simulink model "AutoRS_Simulation"  (R2022b)
settings: Solver=FixedStepAuto  StartTime=0.0  StopTime=350  FixedStep=1/10e3  RelTol=1e-3
undefined symbols (not defined in the file): beta_array, CQ_entries, CT_entries, d_B, d_T, k_B, k_T, lambda_array, m_B, m_T, param_const, param_opt
settings Model: Creator=Aaron  LastModifiedBy=Sebastian
settings DebuggingCC: UnconnectedInputMsg=warning  UnconnectedOutputMsg=warning  UnconnectedLineMsg=warning
settings ModelReferenceCC: EnableRefExpFcnMdlSchedulingChecks=on
settings RTWCC: DLArmComputeVersion=19.05

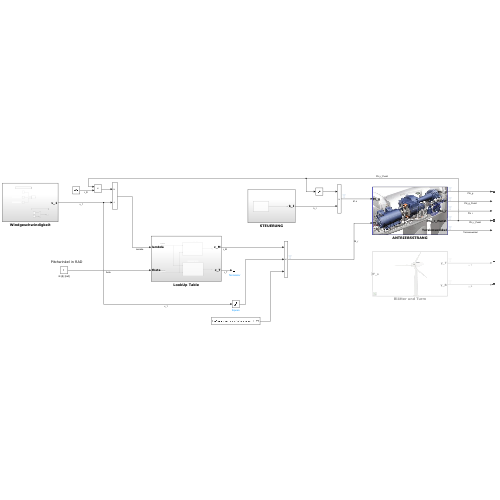
[thumbnail: Simulink's stored preview of the top-level diagram]
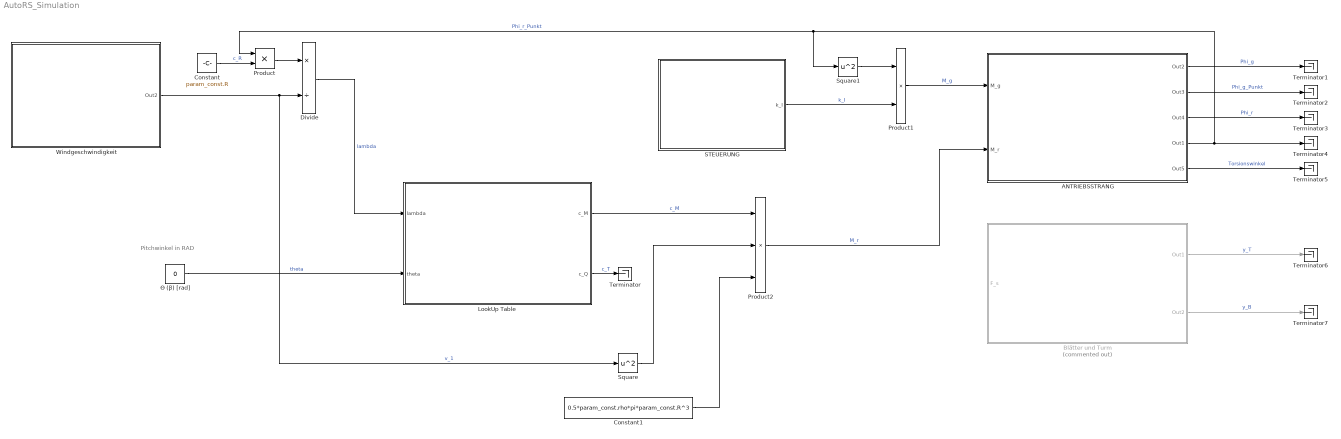
== system AutoRS_Simulation ==
  note: Pitchwinkel in RAD
  ANTRIEBSSTRANG : Subsystem
      mask Display: image('$imagefile'); % Use "Edit Image" on toolstrip to change.
  Blätter und Turm : Subsystem  Commented=on
      mask Display: image('$imagefile'); % Use "Edit Image" on toolstrip to change.
  Constant : Constant  Value=param_const.R
  Constant1 : Constant  Value=0.5*param_const.rho*pi*param_const.R^3
  Divide : Product  Inputs=*/
  LookUp Table : Subsystem
  Product : Product
  Product1 : Product
  Product2 : Product  Inputs=3
  STEUERUNG : Subsystem
  Square : Math  Operator=square
  Square1 : Math  Operator=square
  Terminator{,1..7} (8 alike) : Terminator
  Windgeschwindigkeit : Subsystem
  Θ (β) [rad] : Constant  Value=0
  wires:
  Divide/1 -> LookUp Table/1(lambda)  "lambda"
  Θ (β) [rad]/1 -> LookUp Table/2(theta)  "theta"
  ANTRIEBSSTRANG/1(Out2) -> Terminator1/1  "Phi_g"
  ANTRIEBSSTRANG/2(Out3) -> Terminator2/1  "Phi_g_Punkt"
  ANTRIEBSSTRANG/3(Out4) -> Terminator3/1  "Phi_r"
  ANTRIEBSSTRANG/4(Out1) -> Square1/1, Product/1, Terminator4/1  "Phi_r_Punkt"
  ANTRIEBSSTRANG/5(Out5) -> Terminator5/1  "Torsionswinkel"
  Blätter und Turm/1(Out1) -> Terminator6/1  "y_T"
  Blätter und Turm/2(Out2) -> Terminator7/1  "y_B"
  Product/1 -> Divide/1
  Constant/1 -> Product/2  "c_R"
  Windgeschwindigkeit/1(Out2) -> Square/1, Divide/2  "v_1"
  Product1/1 -> ANTRIEBSSTRANG/1(M_g)  "M_g"
  Product2/1 -> ANTRIEBSSTRANG/2(M_r)  "M_r"
  Square1/1 -> Product1/1
  LookUp Table/2(c_Q) -> Terminator/1  "c_T"
  STEUERUNG/1(k_I) -> Product1/2  "k_I"
  LookUp Table/1(c_M) -> Product2/1  "c_M"
  Square/1 -> Product2/2
  Constant1/1 -> Product2/3

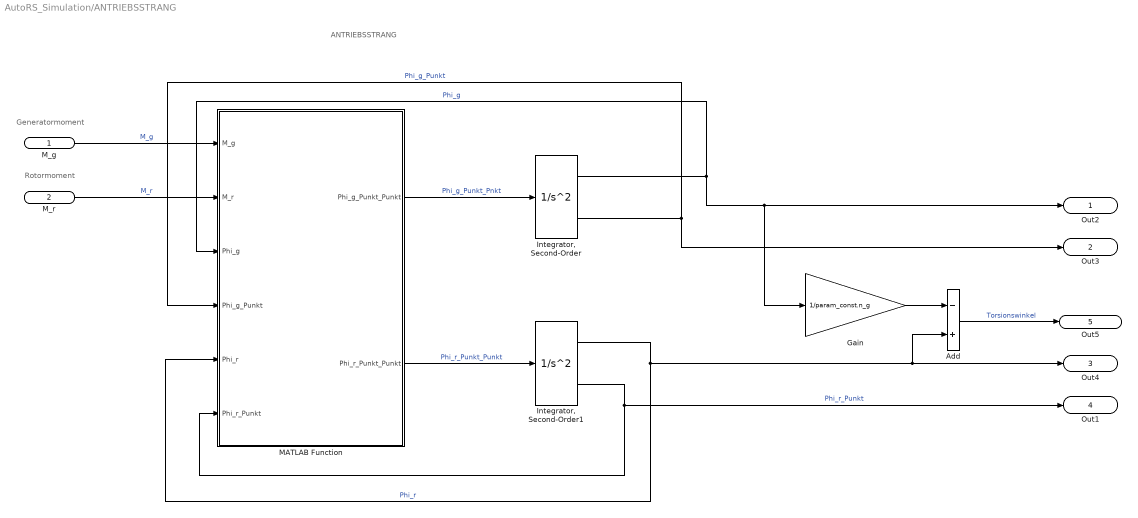
== system AutoRS_Simulation/ANTRIEBSSTRANG ==
  note: ANTRIEBSSTRANG
  note: Rotormoment
  note: Generatormoment
  M_g : Inport
  M_r : Inport  Port=2
  Add : Sum  Inputs=-+
  Gain : Gain  Gain=1/param_const.n_g
  "Integrator, Second-Order" : SecondOrderIntegrator
  "Integrator, Second-Order1" : SecondOrderIntegrator
  MATLAB Function : MATLAB Function  TreatAsAtomicUnit=on
  Out2 : Outport
  Out3 : Outport  Port=2
  Out4 : Outport  Port=3
  Out1 : Outport  Port=4
  Out5 : Outport  Port=5
  wires:
  "Integrator, Second-Order1"/2 -> Out1/1, MATLAB Function/6(Phi_r_Punkt)  "Phi_r_Punkt"
  "Integrator, Second-Order1"/1 -> Out4/1, Add/2, MATLAB Function/5(Phi_r)  "Phi_r"
  MATLAB Function/1(Phi_g_Punkt_Punkt) -> "Integrator, Second-Order"/1  "Phi_g_Punkt_Pnkt"
  "Integrator, Second-Order"/1 -> Out2/1, Gain/1, MATLAB Function/3(Phi_g)  "Phi_g"
  "Integrator, Second-Order"/2 -> Out3/1, MATLAB Function/4(Phi_g_Punkt)  "Phi_g_Punkt"
  Add/1 -> Out5/1  "Torsionswinkel"
  M_g/1 -> MATLAB Function/1(M_g)  "M_g"
  M_r/1 -> MATLAB Function/2(M_r)  "M_r"
  MATLAB Function/2(Phi_r_Punkt_Punkt) -> "Integrator, Second-Order1"/1  "Phi_r_Punkt_Punkt"
  Gain/1 -> Add/1

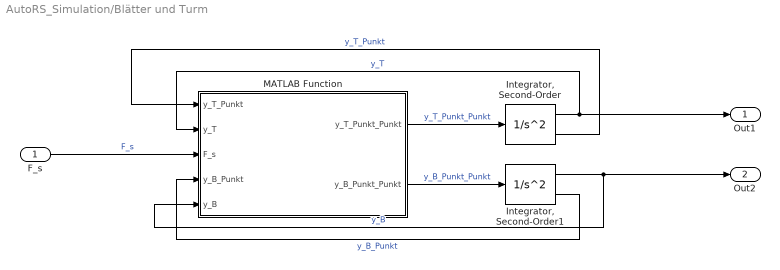
== system AutoRS_Simulation/Blätter und Turm ==
  F_s : Inport
  "Integrator, Second-Order" : SecondOrderIntegrator  ICX=0
  "Integrator, Second-Order1" : SecondOrderIntegrator  ICX=0
  MATLAB Function : MATLAB Function  TreatAsAtomicUnit=on
  Out1 : Outport
  Out2 : Outport  Port=2
  wires:
  MATLAB Function/2(y_B_Punkt_Punkt) -> "Integrator, Second-Order1"/1  "y_B_Punkt_Punkt"
  MATLAB Function/1(y_T_Punkt_Punkt) -> "Integrator, Second-Order"/1  "y_T_Punkt_Punkt"
  "Integrator, Second-Order"/1 -> Out1/1, MATLAB Function/2(y_T)  "y_T"
  F_s/1 -> MATLAB Function/3(F_s)  "F_s"
  "Integrator, Second-Order"/2 -> MATLAB Function/1(y_T_Punkt)  "y_T_Punkt"
  "Integrator, Second-Order1"/2 -> MATLAB Function/4(y_B_Punkt)  "y_B_Punkt"
  "Integrator, Second-Order1"/1 -> Out2/1, MATLAB Function/5(y_B)  "y_B"

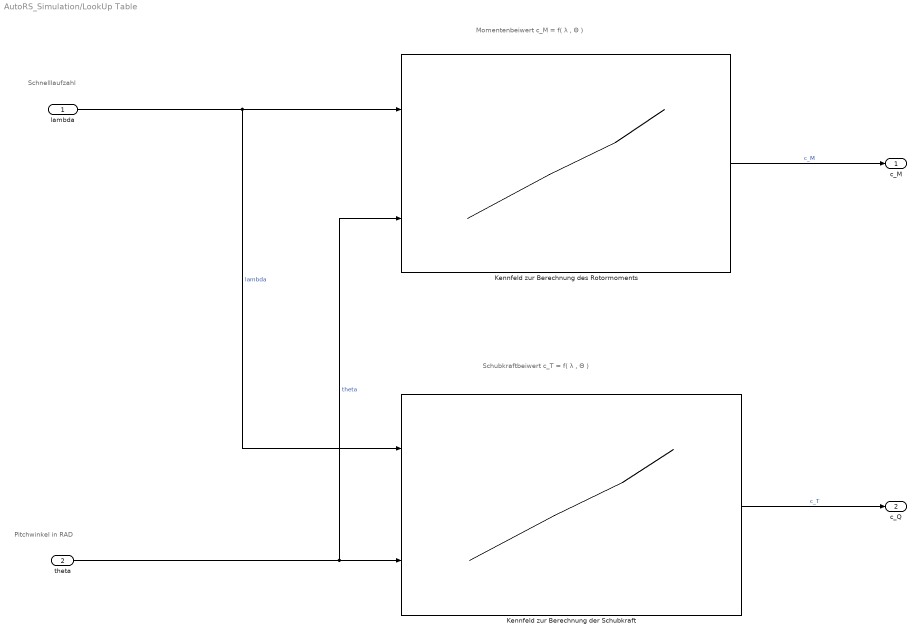
== system AutoRS_Simulation/LookUp Table ==
  note: Schnelllaufzahl
  note: Pitchwinkel in RAD
  note: Momentenbeiwert c_M = f( λ , Θ )
  note: Schubkraftbeiwert c_T = f( λ , Θ )
  lambda : Inport
  theta : Inport  Port=2
  Kennfeld zur Berechnung der Schubkraft : Lookup_n-D  BreakpointsForDimension1=lambda_array  BreakpointsForDimension2=beta_array  Table=CT_entries  InternalRulePriority=Speed  RndMeth=Simplest
      settings: InputPortMap=u0,u1
  Kennfeld zur Berechnung des Rotormoments : Lookup_n-D  BreakpointsForDimension1=lambda_array  BreakpointsForDimension2=beta_array  Table=CQ_entries  InternalRulePriority=Speed  RndMeth=Simplest
      settings: InputPortMap=u0,u1
  c_M : Outport
  c_Q : Outport  Port=2
  wires:
  Kennfeld zur Berechnung der Schubkraft/1 -> c_Q/1  "c_T"
  Kennfeld zur Berechnung des Rotormoments/1 -> c_M/1  "c_M"
  lambda/1 -> Kennfeld zur Berechnung des Rotormoments/1, Kennfeld zur Berechnung der Schubkraft/1  "lambda"
  theta/1 -> Kennfeld zur Berechnung des Rotormoments/2, Kennfeld zur Berechnung der Schubkraft/2  "theta"

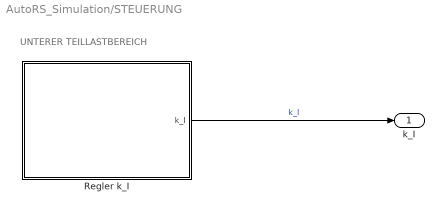
== system AutoRS_Simulation/STEUERUNG ==
  note: UNTERER TEILLASTBEREICH
  Regler k_I : MATLAB Function  TreatAsAtomicUnit=on
  k_I : Outport
  wires:
  Regler k_I/1(k_I) -> k_I/1  "k_I"

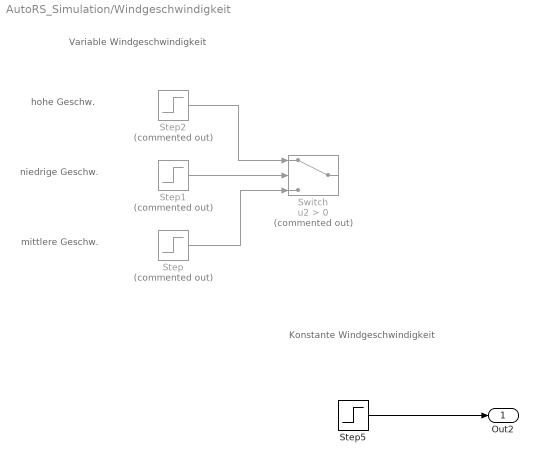
== system AutoRS_Simulation/Windgeschwindigkeit ==
  note: Variable Windgeschwindigkeit
  note: mittlere Geschw.
  note: niedrige Geschw.
  note: hohe Geschw.
  note: Konstante Windgeschwindigkeit
  Step : Step  Commented=on  Time=10  Before=3  After=13  SampleTime=0
  Step1 : Step  Commented=on  Time=20  SampleTime=0
  Step2 : Step  Commented=on  Time=50  Before=13  After=20  SampleTime=0
  Step5 : Step  Time=200  Before=11  SampleTime=0
  Switch : Switch  Commented=on  Criteria=u2 > Threshold  SaturateOnIntegerOverflow=off  InputSameDT=off
  Out2 : Outport
  wires:
  Step2/1 -> Switch/1
  Step/1 -> Switch/3
  Step1/1 -> Switch/2
  Step5/1 -> Out2/1

== matlab function AutoRS_Simulation/Blätter und Turm/MATLAB Function ==
  data: y_T_Punkt input; y_T input; F_s input; y_T_Punkt_Punkt output; y_B_Punkt input; y_B input; y_B_Punkt_Punkt output; k_T parameter; d_T parameter; k_B parameter; d_B parameter; m_T parameter; m_B parameter
function [y_T_Punkt_Punkt, y_B_Punkt_Punkt] = fcn(y_T_Punkt, y_T, F_s, y_B_Punkt, y_B, k_T, d_T, k_B, d_B, m_T, m_B)
    
    % BERECHNUNG
    y_T_Punkt_Punkt = (-k_T*y_T-d_T*y_T_Punkt+3*k_B*(y_B-y_T)+3*d_B*(y_B_Punkt-y_T_Punkt))/m_T;
    
    y_B_Punkt_Punkt = (-3*k_B*(y_B-y_T)-3*d_B*(y_B_Punkt-y_T_Punkt)+F_s)/(3*m_B);
end

== matlab function AutoRS_Simulation/ANTRIEBSSTRANG/MATLAB Function ==
  data: M_g input; M_r input; Phi_g_Punkt_Punkt output; Phi_r_Punkt_Punkt output; Phi_g input; Phi_g_Punkt input; Phi_r input; Phi_r_Punkt input; param_const parameter
function [Phi_g_Punkt_Punkt, Phi_r_Punkt_Punkt]= fcn(M_g, M_r, Phi_g, Phi_g_Punkt, Phi_r, Phi_r_Punkt, param_const)

    % BERECHNUNGEN
    Phi_g_Punkt_Punkt = (-param_const.k_s*(Phi_g-param_const.n_g*Phi_r)-param_const.d_s*(Phi_g_Punkt-param_const.n_g*Phi_r_Punkt)-M_g)/param_const.J_g;

    Phi_r_Punkt_Punkt = (M_r-param_const.n_g*(param_const.k_s*(param_const.n_g*Phi_r-Phi_g))-param_const.n_g*(param_const.d_s*(param_const.n_g*Phi_r_Punkt-Phi_g_Punkt)))/param_const.J_r;
end

== matlab function AutoRS_Simulation/STEUERUNG/Regler k_I ==
  data: k_I output; param_const parameter; param_opt parameter
function k_I = fcn(param_const, param_opt)

    % BERECHNUNG
    k_I = 0.5*param_const.rho*pi*param_const.R^5*(1/param_opt.lambda_opt^3)*(1/param_const.n_g)*param_opt.cP_max;
end
